simulink subsystem "chute_forces"  (R2024b)
settings: Solver=VariableStepAuto  StartTime=0.0  StopTime=10.0  RelTol=1e-3
undefined symbols (not defined in the file or in its folder): chute_drogue_drag, chute_enable, chute_pos_x, time_chute_drogue
settings Model: Creator=finnb  LastModifiedBy=finnb

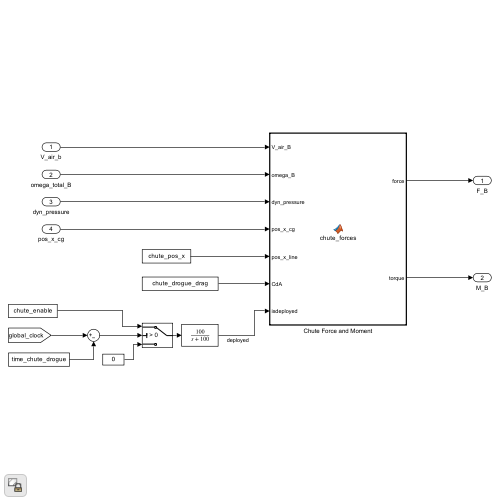
[thumbnail: Simulink's stored preview of the top-level diagram]
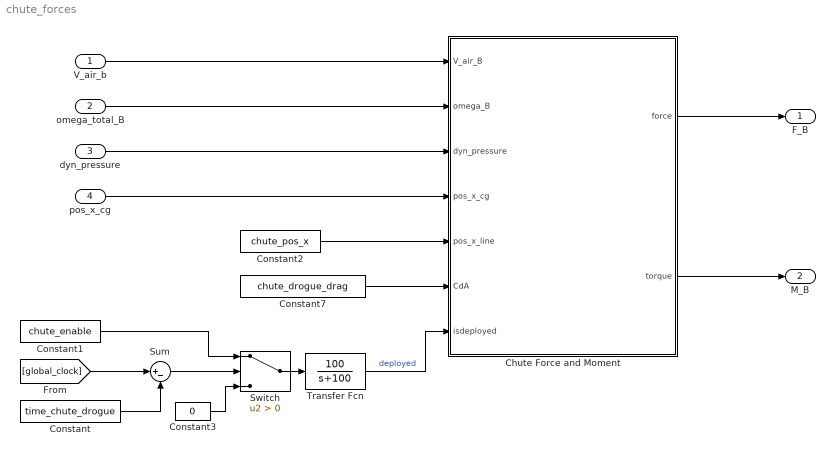
== system chute_forces ==
  V_air_b : Inport
  omega_total_B : Inport  Port=2
  "dyn_pressure " : Inport  Port=3
  pos_x_cg : Inport  Port=4
  Chute Force and Moment : MATLAB Function  TreatAsAtomicUnit=on
  Constant : Constant  Value=time_chute_drogue
  Constant1 : Constant  Value=chute_enable
  Constant2 : Constant  Value=chute_pos_x
  Constant3 : Constant  Value=0
  Constant7 : Constant  Value=chute_drogue_drag
  Sum : Sum  Inputs=|+-
  Switch : Switch  Criteria=u2 > Threshold  SaturateOnIntegerOverflow=off  InputSameDT=off
  Transfer Fcn : TransferFcn  Numerator=[100]  Denominator=[1 100]
  F_B : Outport
  M_B : Outport  Port=2  VectorParamsAs1DForOutWhenUnconnected=off
  wires:
  pos_x_cg/1 -> Chute Force and Moment/4(pos_x_cg)
  Constant2/1 -> Chute Force and Moment/5(pos_x_line)
  Chute Force and Moment/2(torque) -> M_B/1
  V_air_b/1 -> Chute Force and Moment/1(V_air_B)
  omega_total_B/1 -> Chute Force and Moment/2(omega_B)
  Chute Force and Moment/1(force) -> F_B/1
  Constant7/1 -> Chute Force and Moment/6(CdA)
  "dyn_pressure "/1 -> Chute Force and Moment/3(dyn_pressure)
  Constant/1 -> Sum/2
  [global_clock] -> Sum/1
  Sum/1 -> Switch/2
  Switch/1 -> Transfer Fcn/1
  Constant1/1 -> Switch/1
  Constant3/1 -> Switch/3
  Transfer Fcn/1 -> Chute Force and Moment/7(isdeployed)  "deployed"

== matlab function chute_forces/Chute Force and Moment ==
  data: force output; V_air_B input; omega_B input; dyn_pressure input; pos_x_cg input; pos_x_line input; CdA input; torque output; isdeployed input
function [force, torque] = chute_forces(V_air_B, omega_B, dyn_pressure, pos_x_cg, pos_x_line, CdA, isdeployed)

    % moment arm
    pos_x = (pos_x_line - pos_x_cg) * [1;0;0];

    % relative velocity
    Vrel = V_air_B;
    Vrel = V_air_B - cross(omega_B, pos_x);

    % Velocity direction
    V_dir = Vrel / (norm(Vrel) + 1e-10);
    
    %%% Forces  
    % Calculating total force
    F = min(CdA * dyn_pressure, 1000);
    force = - V_dir * F * isdeployed;

    % Total torque
    torque = cross(force, pos_x);

end
